simulink model "zrf_volt_1ant_8bit"  (R2019a)
settings: Solver=VariableStepAuto  StartTime=0.0  StopTime=10.0  RelTol=1e-3
undefined symbols (not defined in the file or in its folder): fft_stages
libraries: xbsIndex_r4 x8883, casper_library_misc x68, xps_library x15, casper_library_sources x8, casper_library_delays x2, casper_library_scopes x2
(part 2 of 97)

== system zrf_volt_1ant_8bit/HTG_ZRF16 ==

== system zrf_volt_1ant_8bit/adc_rstn ==
  convert1_1 : DataTypeConversion  OutDataTypeStr=fixdt('ufix1_En0')  LockScale=on
  convert2_1 : DataTypeConversion  OutDataTypeStr=fixdt('ufix1_En0')  ConvertRealWorld=Stored Integer (SI)  LockScale=on
  gain_1 : Gain
  io_delay : xbsIndex_r4/Delay  rst=off  infoeditControl=Selection of Reset will increase slice count due to use of real FFs and instead of SRLs  en=off  latency=0  reg_retiming=on  dbl_ovrd=off  block_type=delay
  sim_1 : Constant  Value=0
  slice_reg : xbsIndex_r4/Slice  nbits=1  boolean_output=on  mode=Lower Bit Location + Width  bit1=0  base1=MSB of Input  bit0=0  base0=LSB of Input  dbl_ovrd=off  block_type=slice
  zrf_volt_1ant_8bit_adc_rstn_user_data_out : xbsIndex_r4/Gateway In  gui_display_data_type=Fixed-point  arith_type=Unsigned  n_bits=32  bin_pt=0  preci_type=Single  exp_width=8  frac_width=24  rows=1  columns=1  quantization="Round  (unbiased: +/- Inf)"  overflow=Saturate  period=1  UseAsADC=off  ADCChannel='1'  interface=None  automatic_assignment=on  address_offset=hex2dec('00')  intf_name=''  intf_description=''  default_value=0  timing_constraint=None  locs_specified=off  LOCs={}  io_standard={}  inherit_from_input=off  hdl_port=on  dbl_ovrd=off  block_type=gatewayin
  in_reg : Outport
  wires:
  zrf_volt_1ant_8bit_adc_rstn_user_data_out/1 -> io_delay/1
  sim_1/1 -> convert1_1/1
  convert1_1/1 -> convert2_1/1
  convert2_1/1 -> gain_1/1
  gain_1/1 -> zrf_volt_1ant_8bit_adc_rstn_user_data_out/1
  io_delay/1 -> slice_reg/1
  slice_reg/1 -> in_reg/1

== system zrf_volt_1ant_8bit/byte_flip ==
  din : Inport
  join : Subsystem  AncestorBlock=casper_library_flow_control/bus_create  mask(bus_create){inputNum=64}
      mask prompts: inputNum "Number of inputs:"
      mask init:
      | bus_create_init(gcb,...
      |     'inputNum', inputNum);
  reinterpret : xbsIndex_r4/Reinterpret  force_arith_type=on  arith_type=Unsigned  force_bin_pt=on  bin_pt=0  block_type=reinterpret
  reinterpret_out : xbsIndex_r4/Reinterpret  force_arith_type=on  arith_type=Unsigned  force_bin_pt=on  bin_pt=0  block_type=reinterpret
  split : Subsystem  AncestorBlock=casper_library_flow_control/bus_expand  mask(bus_expand){mode=divisions of arbitrary size, outputNum=1, outputWidth=[8 8 8 8 8 8 8 8 8 8 8 8 8 8 8 8 8 8 8 8 8 8 8 8 8 8 8 8 8 8 8 8 8 8 8 8 8 8 8 8 8 8 8 8 8 8 8 8 8 8 8 8 8 8 8 8 8 8 8 8 8 8 8 8], outputBinaryPt=[0 0 0 0 0 0 0 0 0 0 0 0 0 0 0 0 0 0 0 0 0 0 0 0 0 0 0 0 0 0 0 0 0 0 0 0 0 0 0 0 0 0 0 0 0 0 0 0 0 0 0 0 0 0 0 0 0 0 0 0 0 0 0 0], outputArithmeticType=[0 0 0 0 0 0 0 0 0 0 0 0 0 0 0 0 0 0 0 0 0 0 0 0 0 0 0 0 0 0 0 0 0 0 0 0 0 0 0 0 0 0 0 0 0 0 0 0 0 0 0 0 0 0 0 0 0 0 0 0 0 0 0 0], show_format=off, outputToWorkspace=off, variablePrefix=out, outputToModelAsWell=on}
      mask prompts: outputNum "Number of outputs:"; outputWidth "Output width [msb ... lsb]:"; outputBinaryPt "Output binary point position [msb ... lsb]:"; outputArithmeticType "Output arithmetic type (ufix=0, fix=1, bool=2) [msb ... lsb]:"; show_format "Print format string?"; outputToWorkspace "Output to workspace?"; variablePrefix "Variable name prefix:"; outputToModelAsWell "Output to model as well?"
      mask help:
      | Expands a 'bus' made using a bus_create or Xilinx
      | concat block.
      | The input will be divided into the specified number
      | of outputs with the specified arithmetic types.
      | Divisions are made from most significant bit.
      mask init:
      | bus_expand_init(gcb,...
      |     'mode', mode, ...
      |     'outputNum', outputNum, ...
      |     'outputWidth', outputWidth, ...
      |     'outputBinaryPt', outputBinaryPt, ...
      |     'outputArithmeticType', outputArithmeticType, ...
      |     'show_format', show_format, ...
      |     'outputToWorkspace', outputToWorkspace, ...
      |     'variablePrefix', variablePrefix, ...
      |     'outputToModelAsWell', outputToModelAsWell);
      settings: AttributesFormatString=64 outputs
      mask TypeOptions mode: divisions of equal size | divisions of arbitrary size
      mask Callback mode: bus_expand_callback();
      mask Callback outputWidth: bus_expand_callback();
      mask Callback outputToWorkspace: bus_expand_callback();
  dout : Outport
  wires:
  reinterpret_out/1 -> dout/1
  din/1 -> reinterpret/1
  reinterpret/1 -> split/1(bus_in)
  join/1(bus_out) -> reinterpret_out/1
  split/64(lsb_out1) -> join/1(in1)
  split/63(out2) -> join/2(in2)
  split/62(out3) -> join/3(in3)
  split/61(out4) -> join/4(in4)
  split/60(out5) -> join/5(in5)
  split/59(out6) -> join/6(in6)
  split/58(out7) -> join/7(in7)
  split/57(out8) -> join/8(in8)
  split/56(out9) -> join/9(in9)
  split/55(out10) -> join/10(in10)
  split/54(out11) -> join/11(in11)
  split/53(out12) -> join/12(in12)
  split/52(out13) -> join/13(in13)
  split/51(out14) -> join/14(in14)
  split/50(out15) -> join/15(in15)
  split/49(out16) -> join/16(in16)
  split/48(out17) -> join/17(in17)
  split/47(out18) -> join/18(in18)
  split/46(out19) -> join/19(in19)
  split/45(out20) -> join/20(in20)
  split/44(out21) -> join/21(in21)
  split/43(out22) -> join/22(in22)
  split/42(out23) -> join/23(in23)
  split/41(out24) -> join/24(in24)
  split/40(out25) -> join/25(in25)
  split/39(out26) -> join/26(in26)
  split/38(out27) -> join/27(in27)
  split/37(out28) -> join/28(in28)
  split/36(out29) -> join/29(in29)
  split/35(out30) -> join/30(in30)
  split/34(out31) -> join/31(in31)
  split/33(out32) -> join/32(in32)
  split/32(out33) -> join/33(in33)
  split/31(out34) -> join/34(in34)
  split/30(out35) -> join/35(in35)
  split/29(out36) -> join/36(in36)
  split/28(out37) -> join/37(in37)
  split/27(out38) -> join/38(in38)
  split/26(out39) -> join/39(in39)
  split/25(out40) -> join/40(in40)
  split/24(out41) -> join/41(in41)
  split/23(out42) -> join/42(in42)
  split/22(out43) -> join/43(in43)
  split/21(out44) -> join/44(in44)
  split/20(out45) -> join/45(in45)
  split/19(out46) -> join/46(in46)
  split/18(out47) -> join/47(in47)
  split/17(out48) -> join/48(in48)
  split/16(out49) -> join/49(in49)
  split/15(out50) -> join/50(in50)
  split/14(out51) -> join/51(in51)
  split/13(out52) -> join/52(in52)
  split/12(out53) -> join/53(in53)
  split/11(out54) -> join/54(in54)
  split/10(out55) -> join/55(in55)
  split/9(out56) -> join/56(in56)
  split/8(out57) -> join/57(in57)
  split/7(out58) -> join/58(in58)
  split/6(out59) -> join/59(in59)
  split/5(out60) -> join/60(in60)
  split/4(out61) -> join/61(in61)
  split/3(out62) -> join/62(in62)
  split/2(out63) -> join/63(in63)
  split/1(msb_out64) -> join/64(in64)

== system zrf_volt_1ant_8bit/byte_flip1 ==
  din : Inport
  join : Subsystem  AncestorBlock=casper_library_flow_control/bus_create  mask(bus_create){inputNum=64}
      mask prompts: inputNum "Number of inputs:"
      mask init:
      | bus_create_init(gcb,...
      |     'inputNum', inputNum);
  reinterpret : xbsIndex_r4/Reinterpret  force_arith_type=on  arith_type=Unsigned  force_bin_pt=on  bin_pt=0  block_type=reinterpret
  reinterpret_out : xbsIndex_r4/Reinterpret  force_arith_type=on  arith_type=Unsigned  force_bin_pt=on  bin_pt=0  block_type=reinterpret
  split : Subsystem  AncestorBlock=casper_library_flow_control/bus_expand  mask(bus_expand){mode=divisions of arbitrary size, outputNum=1, outputWidth=[8 8 8 8 8 8 8 8 8 8 8 8 8 8 8 8 8 8 8 8 8 8 8 8 8 8 8 8 8 8 8 8 8 8 8 8 8 8 8 8 8 8 8 8 8 8 8 8 8 8 8 8 8 8 8 8 8 8 8 8 8 8 8 8], outputBinaryPt=[0 0 0 0 0 0 0 0 0 0 0 0 0 0 0 0 0 0 0 0 0 0 0 0 0 0 0 0 0 0 0 0 0 0 0 0 0 0 0 0 0 0 0 0 0 0 0 0 0 0 0 0 0 0 0 0 0 0 0 0 0 0 0 0], outputArithmeticType=[0 0 0 0 0 0 0 0 0 0 0 0 0 0 0 0 0 0 0 0 0 0 0 0 0 0 0 0 0 0 0 0 0 0 0 0 0 0 0 0 0 0 0 0 0 0 0 0 0 0 0 0 0 0 0 0 0 0 0 0 0 0 0 0], show_format=off, outputToWorkspace=off, variablePrefix=out, outputToModelAsWell=on}
      mask prompts: outputNum "Number of outputs:"; outputWidth "Output width [msb ... lsb]:"; outputBinaryPt "Output binary point position [msb ... lsb]:"; outputArithmeticType "Output arithmetic type (ufix=0, fix=1, bool=2) [msb ... lsb]:"; show_format "Print format string?"; outputToWorkspace "Output to workspace?"; variablePrefix "Variable name prefix:"; outputToModelAsWell "Output to model as well?"
      mask help:
      | Expands a 'bus' made using a bus_create or Xilinx
      | concat block.
      | The input will be divided into the specified number
      | of outputs with the specified arithmetic types.
      | Divisions are made from most significant bit.
      mask init: same as zrf_volt_1ant_8bit/byte_flip/split
      settings: AttributesFormatString=64 outputs
      mask TypeOptions mode: divisions of equal size | divisions of arbitrary size
      mask Callback mode: bus_expand_callback();
      mask Callback outputWidth: bus_expand_callback();
      mask Callback outputToWorkspace: bus_expand_callback();
  dout : Outport
  wires:
  split/1(msb_out64) -> join/64(in64)
  split/2(out63) -> join/63(in63)
  split/3(out62) -> join/62(in62)
  split/4(out61) -> join/61(in61)
  split/5(out60) -> join/60(in60)
  split/6(out59) -> join/59(in59)
  split/7(out58) -> join/58(in58)
  split/8(out57) -> join/57(in57)
  split/9(out56) -> join/56(in56)
  split/10(out55) -> join/55(in55)
  split/11(out54) -> join/54(in54)
  split/12(out53) -> join/53(in53)
  split/13(out52) -> join/52(in52)
  split/14(out51) -> join/51(in51)
  split/15(out50) -> join/50(in50)
  split/16(out49) -> join/49(in49)
  split/17(out48) -> join/48(in48)
  split/18(out47) -> join/47(in47)
  split/19(out46) -> join/46(in46)
  split/20(out45) -> join/45(in45)
  split/21(out44) -> join/44(in44)
  split/22(out43) -> join/43(in43)
  split/23(out42) -> join/42(in42)
  split/24(out41) -> join/41(in41)
  split/25(out40) -> join/40(in40)
  split/26(out39) -> join/39(in39)
  split/27(out38) -> join/38(in38)
  split/28(out37) -> join/37(in37)
  split/29(out36) -> join/36(in36)
  split/30(out35) -> join/35(in35)
  split/31(out34) -> join/34(in34)
  split/32(out33) -> join/33(in33)
  split/33(out32) -> join/32(in32)
  split/34(out31) -> join/31(in31)
  split/35(out30) -> join/30(in30)
  split/36(out29) -> join/29(in29)
  split/37(out28) -> join/28(in28)
  split/38(out27) -> join/27(in27)
  split/39(out26) -> join/26(in26)
  split/40(out25) -> join/25(in25)
  split/41(out24) -> join/24(in24)
  split/42(out23) -> join/23(in23)
  split/43(out22) -> join/22(in22)
  split/44(out21) -> join/21(in21)
  split/45(out20) -> join/20(in20)
  split/46(out19) -> join/19(in19)
  split/47(out18) -> join/18(in18)
  split/48(out17) -> join/17(in17)
  split/49(out16) -> join/16(in16)
  split/50(out15) -> join/15(in15)
  split/51(out14) -> join/14(in14)
  split/52(out13) -> join/13(in13)
  split/53(out12) -> join/12(in12)
  split/54(out11) -> join/11(in11)
  split/55(out10) -> join/10(in10)
  split/56(out9) -> join/9(in9)
  split/57(out8) -> join/8(in8)
  split/58(out7) -> join/7(in7)
  split/59(out6) -> join/6(in6)
  split/60(out5) -> join/5(in5)
  split/61(out4) -> join/4(in4)
  split/62(out3) -> join/3(in3)
  split/63(out2) -> join/2(in2)
  split/64(lsb_out1) -> join/1(in1)
  join/1(bus_out) -> reinterpret_out/1
  reinterpret/1 -> split/1(bus_in)
  din/1 -> reinterpret/1
  reinterpret_out/1 -> dout/1

== system zrf_volt_1ant_8bit/chan_reorder0 ==
  note: MANUALLY CHANGE BUFFER TO ULTRARAM
  note: output:
      | 4 ants x 2048 chans x [16 time x 2 pols]
      |
      | 8k clocks for complete cycle
  note: Use this programmable
      | map to mess with the channel
      | ordering.
      |
      | This lets us interleave channels we want to send, with channels
      | we don't care about, allowing the data rate to be kept below 10Gb/s
      |
      | Input is 4 channels x 2 pols in parallel.
      | Over 1024 clocks we get a full spectrum for these inputs.
  note: Reorder each parallel 64 bits to combine polarizations:
      |
      | order is now (for each of 4 antenna streams):
      |
      | serial_chans (512) x parallel_chans (4) x pols (2)
  note: reorder serial channels
      | so channels which we don't care about
      | can be placed in convenient
      | place to facilitate inter-packet gaps
  note: input: 16 times x 128 chans x 4 ants x 16 chans(parallel) x 2 pols
      |
      | output:
      | 4 ants x 128 chans x 16 times x 16 chans (parallel) x 2 pols
  note: Only allow one sync after MRST.
      | This is because we don't know the appropriate
      | reorder orders for non-double-buffered runtime-configuratble
      | reorders
  note: Merge streams into 512 bit bus:
      |
      | order is now:
      |
      | serial_chans (128) x 4 ants x parallel_chans (16) x pols (2)
  sync : Inport
  mrst : Inport  Port=2
  din0 : Inport  Port=3
  din1 : Inport  Port=4
  din2 : Inport  Port=5
  din3 : Inport  Port=6
  Concat : xbsIndex_r4/Concat  num_inputs=4  dbl_ovrd=off  block_type=concat
  Constant4 : xbsIndex_r4/Constant  const=1.0  gui_display_data_type=Boolean  arith_type=Boolean  n_bits=16  bin_pt=14  preci_type=Single  exp_width=8  frac_width=24  explicit_period=on  period=1  equ=P=C  opselect=C  inp2=PCIN>>17  opr=+  inp1=P  carry=CIN  dbl_ovrd=off  block_type=constant
  Inverter : xbsIndex_r4/Inverter  en=off  latency=0  dbl_ovrd=off  block_type=inv
  Logical : xbsIndex_r4/Logical  logical_function=AND  inputs=2  en=off  latency=0  precision=Full  arith_type=Unsigned  n_bits=16  bin_pt=0  align_bp=on  dbl_ovrd=off  block_type=logical
  Register : xbsIndex_r4/Register  init=0  rst=on  en=on  dbl_ovrd=off  block_type=register
  parallel_reorder0 : Subsystem
  parallel_reorder1 : Subsystem
  parallel_reorder2 : Subsystem
  parallel_reorder3 : Subsystem
  reorder2 : Subsystem  AncestorBlock=casper_library_reorder/reorder  mask(reorder){map=reshape(permute(reshape([0:512*16 - 1], 512, 16), [2,1]), 512*16, 1), n_bits=512, n_inputs=1, bram_latency=3, map_latency=1, fanout_latency=0, double_buffer=0, bram_map=on, software_controlled=off}
      mask prompts: map "Output Order:"; n_bits "Data width in"; n_inputs "Number of inputs"; bram_latency "BRAM Latency"; map_latency "Map Latency"; fanout_latency "Fanout latency"; double_buffer "Double Buffer"; bram_map "Use BlockRAM for Map"; software_controlled "Use runtime software control"
      mask init:
      | reorder_init(gcb, ...
      |     'map', map, ...
      |     'n_bits', n_bits, ...
      |     'n_inputs', n_inputs, ...
      |     'bram_latency', bram_latency, ...
      |     'map_latency', map_latency, ...
      |     'fanout_latency', fanout_latency, ...
      |     'double_buffer', double_buffer, ...
      |     'bram_map', bram_map, ...
      |     'software_controlled', software_controlled);
      settings: AttributesFormatString=order=13
      mask Help: eval('xlWeb(''http://casper.berkeley.edu/wiki/Reorder'')')
  skip_c_t_transpose : Subsystem  Tag=xps:sw_reg  AncestorBlock=xps_library/Memory/software_register  mask(swreg){io_dir=From Processor, io_delay=0, init_val=0, sample_period=1, names=reg, bitwidths=1, bin_pts=0, arith_types=0, sim_port=on, show_format=on}
      mask prompts: io_dir "I/O direction"; io_delay "I/O delay"; init_val "Initial Value"; sample_period "Sample period"; names "Bitfield names [msb...lsb]"; bitwidths "Bitfield widths"; bin_pts "Bitfield binary pts"; arith_types "Bitfield types, ufix=0, fix=1, bool=2"; sim_port "Provide sim input/output?"; show_format "Print format string?"
      mask help: A 32-bit software-accessible register. Can be divided into bitfields of varying widths and types using the fields in the block mask.
      mask init:
      | swreg_init(gcb)
      settings: AttributesFormatString=1input:uf1.0 = 1 bits
      mask TypeOptions io_dir: To Processor | From Processor
      mask Callback io_dir:
      | mask_enables = get_param(gcb, 'MaskEnables');
      | mask_names = get_param(gcb, 'MaskNames');
      | if strcmp(get_param(gcb, 'io_dir'), 'To Processor'),
      |     mask_enables{ismember(mask_names, 'sample_period')} = 'off';
      | else
      |     mask_enables{ismember(mask_names, 'sample_period')} = 'on';
      | end
      | set_param(gcb, 'MaskEnables', mask_enables);
      mask DialogControl ParameterTabVar0 Prompt: Setup
  square_transposer : Subsystem  AncestorBlock=casper_library_reorder/square_transposer  mask(square_transposer){n_inputs=2, async=off}
      mask prompts: n_inputs "Number of inputs (2^?):"; async "Aynchronus operation"
      mask init:
      | square_transposer_init(gcb,...
      |     'n_inputs', n_inputs, ...
      |     'async', async);
      settings: AttributesFormatString=n_inputs=2
      mask Help: eval('xlWeb(''http://casper.berkeley.edu/wiki/Square_transposer'')')
  transpose_t_c : Subsystem
  sync_out : Outport
  dout0 : Outport  Port=2
  wires:
  skip_c_t_transpose/1(in_reg) -> transpose_t_c/3(bypass)
  transpose_t_c/2(dout) -> dout0/1
  transpose_t_c/1(sync_out) -> sync_out/1
  reorder2/3(dout0) -> transpose_t_c/2(din)
  reorder2/1(sync_out) -> transpose_t_c/1(sync)
  Inverter/1 -> Logical/1
  Register/1 -> Inverter/1
  mrst/1 -> Register/2
  Constant4/1 -> reorder2/2(en)
  Logical/1 -> square_transposer/1(sync)
  sync/1 -> Register/3, Register/1, Logical/2
  din0/1 -> parallel_reorder0/1(din)
  parallel_reorder3/1(dout) -> square_transposer/5(in3)
  parallel_reorder2/1(dout) -> square_transposer/4(in2)
  parallel_reorder1/1(dout) -> square_transposer/3(in1)
  parallel_reorder0/1(dout) -> square_transposer/2(in0)
  square_transposer/1(sync_out) -> reorder2/1(sync)
  Concat/1 -> reorder2/3(din0)
  din1/1 -> parallel_reorder1/1(din)
  din2/1 -> parallel_reorder2/1(din)
  din3/1 -> parallel_reorder3/1(din)
  square_transposer/5(out3) -> Concat/4
  square_transposer/4(out2) -> Concat/3
  square_transposer/3(out1) -> Concat/2
  square_transposer/2(out0) -> Concat/1

== system zrf_volt_1ant_8bit/chan_reorder1 ==
  note: Merge streams into 512 bit bus:
      |
      | order is now:
      |
      | serial_chans (128) x 4 ants x parallel_chans (16) x pols (2)
  note: Only allow one sync after MRST.
      | This is because we don't know the appropriate
      | reorder orders for non-double-buffered runtime-configuratble
      | reorders
  note: input: 16 times x 128 chans x 4 ants x 16 chans(parallel) x 2 pols
      |
      | output:
      | 4 ants x 128 chans x 16 times x 16 chans (parallel) x 2 pols
  note: reorder serial channels
      | so channels which we don't care about
      | can be placed in convenient
      | place to facilitate inter-packet gaps
  note: Reorder each parallel 64 bits to combine polarizations:
      |
      | order is now (for each of 4 antenna streams):
      |
      | serial_chans (512) x parallel_chans (4) x pols (2)
  note: Use this programmable
      | map to mess with the channel
      | ordering.
      |
      | This lets us interleave channels we want to send, with channels
      | we don't care about, allowing the data rate to be kept below 10Gb/s
      |
      | Input is 4 channels x 2 pols in parallel.
      | Over 1024 clocks we get a full spectrum for these inputs.
  note: output:
      | 4 ants x 2048 chans x [16 time x 2 pols]
      |
      | 8k clocks for complete cycle
  note: MANUALLY CHANGE BUFFER TO ULTRARAM
  sync : Inport
  mrst : Inport  Port=2
  din0 : Inport  Port=3
  din1 : Inport  Port=4
  din2 : Inport  Port=5
  din3 : Inport  Port=6
  Concat : xbsIndex_r4/Concat  num_inputs=4  dbl_ovrd=off  block_type=concat
  Constant4 : xbsIndex_r4/Constant  const=1.0  gui_display_data_type=Boolean  arith_type=Boolean  n_bits=16  bin_pt=14  preci_type=Single  exp_width=8  frac_width=24  explicit_period=on  period=1  equ=P=C  opselect=C  inp2=PCIN>>17  opr=+  inp1=P  carry=CIN  dbl_ovrd=off  block_type=constant
  Inverter : xbsIndex_r4/Inverter  en=off  latency=0  dbl_ovrd=off  block_type=inv
  Logical : xbsIndex_r4/Logical  logical_function=AND  inputs=2  en=off  latency=0  precision=Full  arith_type=Unsigned  n_bits=16  bin_pt=0  align_bp=on  dbl_ovrd=off  block_type=logical
  Register : xbsIndex_r4/Register  init=0  rst=on  en=on  dbl_ovrd=off  block_type=register
  parallel_reorder0 : Subsystem
  parallel_reorder1 : Subsystem
  parallel_reorder2 : Subsystem
  parallel_reorder3 : Subsystem
  reorder2 : Subsystem  AncestorBlock=casper_library_reorder/reorder  mask(reorder){map=reshape(permute(reshape([0:512*16 - 1], 512, 16), [2,1]), 512*16, 1), n_bits=512, n_inputs=1, bram_latency=3, map_latency=1, fanout_latency=0, double_buffer=0, bram_map=on, software_controlled=off}
      mask prompts: map "Output Order:"; n_bits "Data width in"; n_inputs "Number of inputs"; bram_latency "BRAM Latency"; map_latency "Map Latency"; fanout_latency "Fanout latency"; double_buffer "Double Buffer"; bram_map "Use BlockRAM for Map"; software_controlled "Use runtime software control"
      mask init: same as zrf_volt_1ant_8bit/chan_reorder0/reorder2
      settings: AttributesFormatString=order=13
      mask Help: eval('xlWeb(''http://casper.berkeley.edu/wiki/Reorder'')')
  skip_c_t_transpose : Subsystem  Tag=xps:sw_reg  AncestorBlock=xps_library/Memory/software_register  mask(swreg){io_dir=From Processor, io_delay=0, init_val=0, sample_period=1, names=reg, bitwidths=1, bin_pts=0, arith_types=0, sim_port=on, show_format=on}
      mask prompts: io_dir "I/O direction"; io_delay "I/O delay"; init_val "Initial Value"; sample_period "Sample period"; names "Bitfield names [msb...lsb]"; bitwidths "Bitfield widths"; bin_pts "Bitfield binary pts"; arith_types "Bitfield types, ufix=0, fix=1, bool=2"; sim_port "Provide sim input/output?"; show_format "Print format string?"
      mask help: A 32-bit software-accessible register. Can be divided into bitfields of varying widths and types using the fields in the block mask.
      mask init:
      | swreg_init(gcb)
      settings: AttributesFormatString=1input:uf1.0 = 1 bits
      mask TypeOptions io_dir: To Processor | From Processor
      mask Callback io_dir:
      | mask_enables = get_param(gcb, 'MaskEnables');
      | mask_names = get_param(gcb, 'MaskNames');
      | if strcmp(get_param(gcb, 'io_dir'), 'To Processor'),
      |     mask_enables{ismember(mask_names, 'sample_period')} = 'off';
      | else
      |     mask_enables{ismember(mask_names, 'sample_period')} = 'on';
      | end
      | set_param(gcb, 'MaskEnables', mask_enables);
      mask DialogControl ParameterTabVar0 Prompt: Setup
  square_transposer : Subsystem  AncestorBlock=casper_library_reorder/square_transposer  mask(square_transposer){n_inputs=2, async=off}
      mask prompts: n_inputs "Number of inputs (2^?):"; async "Aynchronus operation"
      mask init:
      | square_transposer_init(gcb,...
      |     'n_inputs', n_inputs, ...
      |     'async', async);
      settings: AttributesFormatString=n_inputs=2
      mask Help: eval('xlWeb(''http://casper.berkeley.edu/wiki/Square_transposer'')')
  transpose_t_c : Subsystem
  sync_out : Outport
  dout0 : Outport  Port=2
  wires:
  square_transposer/2(out0) -> Concat/1
  square_transposer/3(out1) -> Concat/2
  square_transposer/4(out2) -> Concat/3
  square_transposer/5(out3) -> Concat/4
  din3/1 -> parallel_reorder3/1(din)
  din2/1 -> parallel_reorder2/1(din)
  din1/1 -> parallel_reorder1/1(din)
  Concat/1 -> reorder2/3(din0)
  square_transposer/1(sync_out) -> reorder2/1(sync)
  parallel_reorder0/1(dout) -> square_transposer/2(in0)
  parallel_reorder1/1(dout) -> square_transposer/3(in1)
  parallel_reorder2/1(dout) -> square_transposer/4(in2)
  parallel_reorder3/1(dout) -> square_transposer/5(in3)
  din0/1 -> parallel_reorder0/1(din)
  sync/1 -> Logical/2, Register/1, Register/3
  Logical/1 -> square_transposer/1(sync)
  Constant4/1 -> reorder2/2(en)
  mrst/1 -> Register/2
  Register/1 -> Inverter/1
  Inverter/1 -> Logical/1
  reorder2/1(sync_out) -> transpose_t_c/1(sync)
  reorder2/3(dout0) -> transpose_t_c/2(din)
  transpose_t_c/1(sync_out) -> sync_out/1
  transpose_t_c/2(dout) -> dout0/1
  skip_c_t_transpose/1(in_reg) -> transpose_t_c/3(bypass)

== system zrf_volt_1ant_8bit/corr ==
  sync : Inport
  din : Inport  Port=2
  mrst : Inport  Port=3
  bus_create1 : Subsystem  AncestorBlock=casper_library_flow_control/bus_create  mask(bus_create){inputNum=4}
      mask prompts: inputNum "Number of inputs:"
      mask init:
      | bus_create_init(gcb,...
      |     'inputNum', inputNum);
  bus_expand : Subsystem  AncestorBlock=casper_library_flow_control/bus_expand  mask(bus_expand){mode=divisions of equal size, outputNum=2, outputWidth=25*2*4, outputBinaryPt=0, outputArithmeticType=0, show_format=off, outputToWorkspace=off, variablePrefix=out, outputToModelAsWell=on}
      mask prompts: outputNum "Number of outputs:"; outputWidth "Output width:"; outputBinaryPt "Output binary point position:"; outputArithmeticType "Output arithmetic type (ufix=0, fix=1, bool=2):"; show_format "Print format string?"; outputToWorkspace "Output to workspace?"; variablePrefix "Variable name prefix:"; outputToModelAsWell "Output to model as well?"
      mask help:
      | Expands a 'bus' made using a bus_create or Xilinx
      | concat block.
      | The input will be divided into the specified number
      | of outputs with the specified arithmetic types.
      | Divisions are made from most significant bit.
      mask init: same as zrf_volt_1ant_8bit/byte_flip/split
      settings: AttributesFormatString=2 outputs
      mask TypeOptions mode: divisions of equal size | divisions of arbitrary size
      mask Callback mode: bus_expand_callback();
      mask Callback outputWidth: bus_expand_callback();
      mask Callback outputToWorkspace: bus_expand_callback();
  bus_expand3 : Subsystem  AncestorBlock=casper_library_flow_control/bus_expand  mask(bus_expand){mode=divisions of equal size, outputNum=4, outputWidth=25*2, outputBinaryPt=0, outputArithmeticType=0, show_format=off, outputToWorkspace=off, variablePrefix=out, outputToModelAsWell=on}
      mask prompts: outputNum "Number of outputs:"; outputWidth "Output width:"; outputBinaryPt "Output binary point position:"; outputArithmeticType "Output arithmetic type (ufix=0, fix=1, bool=2):"; show_format "Print format string?"; outputToWorkspace "Output to workspace?"; variablePrefix "Variable name prefix:"; outputToModelAsWell "Output to model as well?"
      mask help:
      | Expands a 'bus' made using a bus_create or Xilinx
      | concat block.
      | The input will be divided into the specified number
      | of outputs with the specified arithmetic types.
      | Divisions are made from most significant bit.
      mask init: same as zrf_volt_1ant_8bit/byte_flip/split
      settings: AttributesFormatString=4 outputs
      mask TypeOptions mode: divisions of equal size | divisions of arbitrary size
      mask Callback mode: bus_expand_callback();
      mask Callback outputWidth: bus_expand_callback();
      mask Callback outputToWorkspace: bus_expand_callback();
  bus_expand4 : Subsystem  AncestorBlock=casper_library_flow_control/bus_expand  mask(bus_expand){mode=divisions of equal size, outputNum=4, outputWidth=25*2, outputBinaryPt=0, outputArithmeticType=0, show_format=off, outputToWorkspace=off, variablePrefix=out, outputToModelAsWell=on}
      mask prompts: outputNum "Number of outputs:"; outputWidth "Output width:"; outputBinaryPt "Output binary point position:"; outputArithmeticType "Output arithmetic type (ufix=0, fix=1, bool=2):"; show_format "Print format string?"; outputToWorkspace "Output to workspace?"; variablePrefix "Variable name prefix:"; outputToModelAsWell "Output to model as well?"
      mask help:
      | Expands a 'bus' made using a bus_create or Xilinx
      | concat block.
      | The input will be divided into the specified number
      | of outputs with the specified arithmetic types.
      | Divisions are made from most significant bit.
      mask init: same as zrf_volt_1ant_8bit/byte_flip/split
      settings: AttributesFormatString=4 outputs
      mask TypeOptions mode: divisions of equal size | divisions of arbitrary size
      mask Callback mode: bus_expand_callback();
      mask Callback outputWidth: bus_expand_callback();
      mask Callback outputToWorkspace: bus_expand_callback();
  crosspower_vacc : Subsystem  mask{bw=25, nchan=2^n_chan_bits, vacc_bw=64, vacc_bp=48}
      mask prompts: bw "Bitwidth in"; nchan "Number of channels"; vacc_bw "Vector accumulator output bitwidth"; vacc_bp "Vector accumulator output binary point"
  ss_vld_out : Outport
  ss_dout : Outport  Port=2
  wires:
  din/1 -> bus_expand/1(bus_in)
  bus_expand/1(msb_out2) -> [x]
  bus_expand/2(lsb_out1) -> [y]
  sync/1 -> [sync_in]
  mrst/1 -> [mrst_in]
  crosspower_vacc/2(xy0) -> [xy_0]
  crosspower_vacc/5(xy3) -> [xy_3]
  crosspower_vacc/4(xy2) -> [xy_2]
  crosspower_vacc/3(xy1) -> [xy_1]
  bus_expand3/1(msb_out4) -> crosspower_vacc/2(x0)
  bus_expand3/2(out3) -> crosspower_vacc/3(x1)
  bus_expand3/3(out2) -> crosspower_vacc/4(x2)
  bus_expand3/4(lsb_out1) -> crosspower_vacc/5(x3)
  bus_expand4/1(msb_out4) -> crosspower_vacc/6(y0)
  bus_expand4/2(out3) -> crosspower_vacc/7(y1)
  bus_expand4/3(out2) -> crosspower_vacc/8(y2)
  bus_expand4/4(lsb_out1) -> crosspower_vacc/9(y3)
  [vacc_vld] -> ss_vld_out/1
  bus_create1/1(bus_out) -> ss_dout/1
  [sync_in] -> crosspower_vacc/1(new_acc)
  [x] -> bus_expand3/1(bus_in)
  [y] -> bus_expand4/1(bus_in)
  [xy_0] -> bus_create1/1(in1)
  [xy_1] -> bus_create1/2(in2)
  [xy_2] -> bus_create1/3(in3)
  [xy_3] -> bus_create1/4(in4)
  crosspower_vacc/1(vld) -> [vacc_vld]

== system zrf_volt_1ant_8bit/corr_quant ==
  sync : Inport
  din : Inport  Port=2
  bus_expand : Subsystem  AncestorBlock=casper_library_flow_control/bus_expand  mask(bus_expand){mode=divisions of equal size, outputNum=2, outputWidth=4*2*4, outputBinaryPt=0, outputArithmeticType=0, show_format=off, outputToWorkspace=off, variablePrefix=out, outputToModelAsWell=on}
      mask prompts: outputNum "Number of outputs:"; outputWidth "Output width:"; outputBinaryPt "Output binary point position:"; outputArithmeticType "Output arithmetic type (ufix=0, fix=1, bool=2):"; show_format "Print format string?"; outputToWorkspace "Output to workspace?"; variablePrefix "Variable name prefix:"; outputToModelAsWell "Output to model as well?"
      mask help:
      | Expands a 'bus' made using a bus_create or Xilinx
      | concat block.
      | The input will be divided into the specified number
      | of outputs with the specified arithmetic types.
      | Divisions are made from most significant bit.
      mask init: same as zrf_volt_1ant_8bit/byte_flip/split
      settings: AttributesFormatString=2 outputs
      mask TypeOptions mode: divisions of equal size | divisions of arbitrary size
      mask Callback mode: bus_expand_callback();
      mask Callback outputWidth: bus_expand_callback();
      mask Callback outputToWorkspace: bus_expand_callback();
  bus_expand1 : Subsystem  AncestorBlock=casper_library_flow_control/bus_expand  mask(bus_expand){mode=divisions of equal size, outputNum=4, outputWidth=4*2, outputBinaryPt=0, outputArithmeticType=1, show_format=off, outputToWorkspace=off, variablePrefix=out, outputToModelAsWell=on}
      mask prompts: outputNum "Number of outputs:"; outputWidth "Output width:"; outputBinaryPt "Output binary point position:"; outputArithmeticType "Output arithmetic type (ufix=0, fix=1, bool=2):"; show_format "Print format string?"; outputToWorkspace "Output to workspace?"; variablePrefix "Variable name prefix:"; outputToModelAsWell "Output to model as well?"
      mask help:
      | Expands a 'bus' made using a bus_create or Xilinx
      | concat block.
      | The input will be divided into the specified number
      | of outputs with the specified arithmetic types.
      | Divisions are made from most significant bit.
      mask init: same as zrf_volt_1ant_8bit/byte_flip/split
      settings: AttributesFormatString=4 outputs
      mask TypeOptions mode: divisions of equal size | divisions of arbitrary size
      mask Callback mode: bus_expand_callback();
      mask Callback outputWidth: bus_expand_callback();
      mask Callback outputToWorkspace: bus_expand_callback();
  bus_expand2 : Subsystem  AncestorBlock=casper_library_flow_control/bus_expand  mask(bus_expand){mode=divisions of equal size, outputNum=4, outputWidth=4*2, outputBinaryPt=0, outputArithmeticType=1, show_format=off, outputToWorkspace=off, variablePrefix=out, outputToModelAsWell=on}
      mask prompts: outputNum "Number of outputs:"; outputWidth "Output width:"; outputBinaryPt "Output binary point position:"; outputArithmeticType "Output arithmetic type (ufix=0, fix=1, bool=2):"; show_format "Print format string?"; outputToWorkspace "Output to workspace?"; variablePrefix "Variable name prefix:"; outputToModelAsWell "Output to model as well?"
      mask help:
      | Expands a 'bus' made using a bus_create or Xilinx
      | concat block.
      | The input will be divided into the specified number
      | of outputs with the specified arithmetic types.
      | Divisions are made from most significant bit.
      mask init: same as zrf_volt_1ant_8bit/byte_flip/split
      settings: AttributesFormatString=4 outputs
      mask TypeOptions mode: divisions of equal size | divisions of arbitrary size
      mask Callback mode: bus_expand_callback();
      mask Callback outputWidth: bus_expand_callback();
      mask Callback outputToWorkspace: bus_expand_callback();
  power_vacc0 : Subsystem  mask{bw=8, nchan=2^n_chan_bits, vacc_bw=32, vacc_bp=14}
      mask prompts: bw "Bitwidth in"; nchan "Number of channels"; vacc_bw "Vector accumulator output bitwidth"; vacc_bp "Vector accumulator output binary point"
  power_vacc1 : Subsystem  mask{bw=8, nchan=2^n_chan_bits, vacc_bw=32, vacc_bp=14}
      mask prompts: bw "Bitwidth in"; nchan "Number of channels"; vacc_bw "Vector accumulator output bitwidth"; vacc_bp "Vector accumulator output binary point"
  vacc_ss : Subsystem  mask{n_chan_bits=n_chan_bits}
      mask prompts: n_chan_bits "Number of channels (2^?)"
      mask init:
      | ss0 = [gcb '/ss0']
      | %ss1 = [gcb '/ss1']
      | 
      | nsamples = num2str(n_chan_bits - 2);
      | 
      | set_param(ss0, 'nsamples', nsamples);
      | %set_param(ss1, 'nsamples', nsamples);
  wires:
  bus_expand2/4(lsb_out1) -> power_vacc1/5(in3)
  bus_expand2/3(out2) -> power_vacc1/4(in2)
  bus_expand2/2(out3) -> power_vacc1/3(in1)
  bus_expand2/1(msb_out4) -> power_vacc1/2(in0)
  bus_expand1/4(lsb_out1) -> power_vacc0/5(in3)
  bus_expand1/3(out2) -> power_vacc0/4(in2)
  bus_expand1/2(out3) -> power_vacc0/3(in1)
  bus_expand1/1(msb_out4) -> power_vacc0/2(in0)
  [yy_3] -> vacc_ss/9(yy3)
  [yy_2] -> vacc_ss/8(yy2)
  [yy_1] -> vacc_ss/7(yy1)
  [yy_0] -> vacc_ss/6(yy0)
  [xx_3] -> vacc_ss/5(xx3)
  [xx_2] -> vacc_ss/4(xx2)
  power_vacc1/5(out3) -> [yy_3]
  power_vacc1/4(out2) -> [yy_2]
  power_vacc1/3(out1) -> [yy_1]
  power_vacc1/2(out0) -> [yy_0]
  power_vacc0/5(out3) -> [xx_3]
  power_vacc0/4(out2) -> [xx_2]
  power_vacc0/3(out1) -> [xx_1]
  power_vacc0/2(out0) -> [xx_0]
  [xx_1] -> vacc_ss/3(xx1)
  [vacc_vld] -> vacc_ss/1(vld)
  [xx_0] -> vacc_ss/2(xx0)
  [y] -> bus_expand2/1(bus_in)
  sync/1 -> [sync_in]
  [sync_in] -> power_vacc1/1(new_acc)
  [x] -> bus_expand1/1(bus_in)
  bus_expand/2(lsb_out1) -> [y]
  bus_expand/1(msb_out2) -> [x]
  din/1 -> bus_expand/1(bus_in)
  power_vacc0/1(vld) -> [vacc_vld]
  [sync_in] -> power_vacc0/1(new_acc)

== system zrf_volt_1ant_8bit/edge_detect ==
  in : Inport
  Delay : xbsIndex_r4/Delay  rst=off  infoeditControl=Selection of Reset will increase slice count due to use of real FFs and instead of SRLs  en=off  latency=1  reg_retiming=off  dbl_ovrd=off  block_type=delay
      settings: xl_area=[0, 0, 0, 0, 0, 0, 0]
  Inverter : xbsIndex_r4/Inverter  en=off  latency=0  dbl_ovrd=off  block_type=inv
      settings: xl_area=[0, 0, 0, 0, 0, 0, 0]
  edge_op : xbsIndex_r4/Logical  logical_function=NOR  inputs=2  en=off  latency=0  precision=Full  arith_type=Unsigned  n_bits=8  bin_pt=2  align_bp=on  dbl_ovrd=off  block_type=logical
      settings: xl_area=[0, 0, 0, 0, 0, 0, 0]
  out : Outport
  wires:
  Inverter/1 -> edge_op/1
  edge_op/1 -> out/1
  in/1 -> Inverter/1, Delay/1
  Delay/1 -> edge_op/2

== system zrf_volt_1ant_8bit/eth0 ==
  data : Inport
  vld : Inport  Port=2
  eof : Inport  Port=3
  dest_ip : Inport  Port=4
  dest_port : Inport  Port=5
  byte_enable : Inport  Port=6
  Constant : xbsIndex_r4/Constant  const=0  gui_display_data_type=Boolean  arith_type=Boolean  n_bits=1  bin_pt=0  preci_type=Single  exp_width=8  frac_width=24  explicit_period=on  period=1  equ=P=C  opselect=C  inp2=PCIN>>17  opr=+  inp1=P  carry=CIN  dbl_ovrd=off  block_type=constant
  Constant1 : xbsIndex_r4/Constant  const=0  gui_display_data_type=Boolean  arith_type=Boolean  n_bits=1  bin_pt=0  preci_type=Single  exp_width=8  frac_width=24  explicit_period=on  period=1  equ=P=C  opselect=C  inp2=PCIN>>17  opr=+  inp1=P  carry=CIN  dbl_ovrd=off  block_type=constant
  Constant2 : xbsIndex_r4/Constant  const=1  gui_display_data_type=Fixed-point  arith_type=Unsigned  n_bits=1  bin_pt=0  preci_type=Single  exp_width=8  frac_width=24  explicit_period=on  period=1  equ=P=C  opselect=C  inp2=PCIN>>17  opr=+  inp1=P  carry=CIN  dbl_ovrd=off  block_type=constant
  Constant3 : xbsIndex_r4/Constant  const=0  gui_display_data_type=Fixed-point  arith_type=Unsigned  n_bits=1  bin_pt=0  preci_type=Single  exp_width=8  frac_width=24  explicit_period=on  period=1  equ=P=C  opselect=C  inp2=PCIN>>17  opr=+  inp1=P  carry=CIN  dbl_ovrd=off  block_type=constant
  Delay : xbsIndex_r4/Delay  rst=off  infoeditControl=Selection of Reset will increase slice count due to use of real FFs and instead of SRLs  en=off  latency=1  reg_retiming=off  dbl_ovrd=off  block_type=delay
  Logical : xbsIndex_r4/Logical  logical_function=AND  inputs=2  en=off  latency=0  precision=Full  arith_type=Unsigned  n_bits=16  bin_pt=0  align_bp=on  dbl_ovrd=off  block_type=logical
  Register : xbsIndex_r4/Register  init=0  rst=off  en=on  dbl_ovrd=off  block_type=register
  Slice : xbsIndex_r4/Slice  nbits=1  boolean_output=on  mode=Lower Bit Location + Width  bit1=0  base1=MSB of Input  bit0=0  base0=LSB of Input  dbl_ovrd=off  block_type=slice
  Slice1 : xbsIndex_r4/Slice  nbits=1  boolean_output=on  mode=Lower Bit Location + Width  bit1=0  base1=MSB of Input  bit0=1  base0=LSB of Input  dbl_ovrd=off  block_type=slice
  Slice2 : xbsIndex_r4/Slice  nbits=16  boolean_output=off  mode=Lower Bit Location + Width  bit1=0  base1=MSB of Input  bit0=2  base0=LSB of Input  dbl_ovrd=off  block_type=slice
  Slice3 : xbsIndex_r4/Slice  nbits=1  boolean_output=on  mode=Lower Bit Location + Width  bit1=0  base1=MSB of Input  bit0=2+16  base0=LSB of Input  dbl_ovrd=off  block_type=slice
  ctrl : Subsystem  Tag=xps:sw_reg  AncestorBlock=xps_library/Memory/software_register  mask(swreg){io_dir=From Processor, io_delay=0, init_val=0, sample_period=1, names=reg, bitwidths=32, bin_pts=0, arith_types=0, sim_port=on, show_format=off}
      mask prompts: io_dir "I/O direction"; io_delay "I/O delay"; init_val "Initial Value"; sample_period "Sample period"; names "Bitfield names [msb...lsb]"; bitwidths "Bitfield widths"; bin_pts "Bitfield binary pts"; arith_types "Bitfield types, ufix=0, fix=1, bool=2"; sim_port "Provide sim input/output?"; show_format "Print format string?"
      mask help: A 32-bit software-accessible register. Can be divided into bitfields of varying widths and types using the fields in the block mask.
      mask init:
      | swreg_init(gcb)
      settings: AttributesFormatString=1input
      mask TypeOptions io_dir: To Processor | From Processor
      mask Callback io_dir:
      | mask_enables = get_param(gcb, 'MaskEnables');
      | mask_names = get_param(gcb, 'MaskNames');
      | if strcmp(get_param(gcb, 'io_dir'), 'To Processor'),
      |     mask_enables{ismember(mask_names, 'sample_period')} = 'off';
      | else
      |     mask_enables{ismember(mask_names, 'sample_period')} = 'on';
      | end
      | set_param(gcb, 'MaskEnables', mask_enables);
      mask DialogControl ParameterTabVar0 Prompt: Setup
  lpmode_gpio : xps_library/IO/gpio  Tag=xps:gpio  io_group_params_forwarded=off  io_group=ROACH:led  io_group_real=custom  io_group_custom=qsfp_lpmode  io_dir=out  arith_type=Unsigned  bitwidth=1  bin_pt=0  bit_index=[0]  sample_period=1  use_single_ended=off  use_ddr=off  reg_iob=on  reg_clk_phase=0  termination=None
      settings: SourceProductName=CASPER XPS Blockset
  onehundred_gbe : Subsystem  Tag=xps:onehundred_gbe  AncestorBlock=xps_library/IO/onehundred_gbe  mask(forty_gbe){flavour=cx4, slot=1, port_r1=0, port_r2_cx4=0, port_r2_sfpp=0, port=0, rx_dist_ram=on, large_frames=on, input_pipeline_delay=0, show_param=on, pre_emph_r2=0.74, pre_emph=3, post_emph_r2=0.18, rxeqmix_r2=7, swing_r2=940, swing=800, fab_en=on, fab_mac=hex2dec('123456780000'), fab_ip=192*(2^24) + 168*(2^16) + 5*(2^8) + 20*(2^0), fab_udp=10000, fab_gate=1, cpu_rx_en=on, cpu_tx_en=on, ttl=hex2dec('FF'), promisc_mode=off, debug_ctr_width=16, debug_en_all=off, debug_dis_all=off, txctr=off, txerrctr=off, txerrctr_len=100, txofctr=off, txfullctr=off, txvldctr=off, txsnaplen=0 - no snap, rxctr=off, rxerrctr=off, rxerrctr_len=100, rxofctr=off, rxbadctr=off, rxvldctr=off, rxeofctr=off, rxsnaplen=0 - no snap, rxsrcip=off, rxdstip=off}
      mask prompts: flavour "Mezzanine card flavour"; slot "Card slot"; port_r1 "Port"; port_r2_cx4 "Port"; port_r2_sfpp "Port"; rx_dist_ram "Shallow RX Fifo (Beware overruns!)"; large_frames "Enable Large TX Frames (8k+512)"; input_pipeline_delay "Incoming pipeline delay"; show_param "---------------------- Show Implementation Parameters -----------------------------------------------------------------------------------"; pre_emph_r2 "Pre-emphasis (dB)"; pre_emph "Pre-emphasis"; post_emph_r2 "Post-emphasis (dB)"; rxeqmix_r2 "Receive equalisation"; swing_r2 "Driver Swing Control (mVppd)"; swing "Differential swing"; fab_en "Enable fabric on startup"; fab_mac "Fabric MAC Address"; fab_ip "Fabric IP Address"; fab_udp "Fabric UDP Port"; fab_gate "Fabric Gateway"; cpu_rx_en "Enable CPU RX"; cpu_tx_en "Enable CPU TX"; promisc_mode "Promiscuous mode"; debug_ctr_width "Debug counter width"; debug_en_all "Enable all counters (overrides individual settings)"; debug_dis_all "Disable all counters (overrides individual settings)"; txctr "TX - core_txctr"; txerrctr "TX packet length error - core_txerrctr"; txerrctr_len "-- expected TX packet length"; txofctr "TX overflow - core_txofctr"; txfullctr "TX full - core_txfullctr"; txvldctr "TX valid cycle - core_txvldctr"; txsnaplen "TX snapshot length"; rxctr "RX - core_rxctr"; rxerrctr "RX packet length error - core_rxerrctr"; rxerrctr_len "-- expected RX packet length"; rxofctr "RX overflow - core_rxofctr"; rxbadctr "RX bad - core_rxbadctr"; rxvldctr "RX valid cycle - core_rxvldctr"; rxeofctr "RX eof - core_rxeofctr"; rxsnaplen "RX snapshot length"; rxsrcip "RX snapshot - include source IPs"; rxdstip "RX snapshot - include destination IPs"
      mask help: This block sends and receives UDP frames (packets). It accepts a 64 bit wide data stream with user-determined frame breaks. The data stream is wrapped in a UDP frame for transmission. Incoming UDP packets are unwrapped and the data presented as a 64 bit wide stream.
      mask init:
      | temp = eval(get_param(gcb, 'debug_ctr_width'));
      | if temp <= 0,
      |     error('Debug counters cannot be <= zero.');
      | end
      | onehundred_gbe_mask(gcb)
      settings: AttributesFormatString=incoming_latency=0
      mask TypeOptions flavour: sfp+ | cx4
      mask Callback flavour: forty_gbe_callback
      mask TypeOptions slot: 0 | 1
      mask TypeOptions port_r1: 0 | 1 | 2 | 3
      mask TypeOptions port_r2_cx4: 0 | 1 | 2
      mask TypeOptions port_r2_sfpp: 0 | 1 | 2 | 3
      mask TypeOptions port: 0 | 1 | 2 | 3
      mask Callback show_param: forty_gbe_callback
      mask TypeOptions pre_emph_r2: 0.15 | 0.3 | 0.45 | 0.61 | 0.74 | 0.91 | 1.07 | 1.25 | 1.36 | 1.55 | 1.74 | 1.94 | 2.11 | 2.32 | 2.54 | 2.77
      mask TypeOptions pre_emph: 0 | 1 | 2 | 3
      mask TypeOptions post_emph_r2: 0.18 | 0.19 | 0.2 | 0.39 | 0.63 | 0.82 | 1.07 | 1.32 | 1.6 | 1.65 | 1.94 | 2.21 | 2.52 | 2.76 | 3.08 | 3.41 | 3.77 | 3.97 | 4.36 | 4.73 | 5.16 | 5.47 | 5.93 | 6.38 | 6.89
      mask TypeOptions rxeqmix_r2: 0 | 1 | 2 | 3 | 4 | 5 | 6 | 7
      mask TypeOptions swing_r2: 110 | 210 | 310 | 400 | 480 | 570 | 660 | 740 | 810 | 880 | 940 | 990 | 1040 | 1080 | 1110 | 1130
      mask TypeOptions swing: 400 | 500 | 600 | 700 | 800
      mask Callback debug_en_all:
      | if strcmp(get_param(gcb, 'debug_en_all'), 'on')
      |     set_param(gcb, 'debug_dis_all', 'off')
      | end
      mask Callback debug_dis_all:
      | if strcmp(get_param(gcb, 'debug_dis_all'), 'on')
      |     set_param(gcb, 'debug_en_all', 'off')
      | end
      mask Callback txerrctr:
      | blk = gcb;
      | mask_visibilities = get_param(blk, 'MaskVisibilities');
      | mask_names = get_param(blk, 'MaskNames');
      | if strcmp(get_param(blk, 'txerrctr'), 'on')
      |     mask_visibilities{ismember(mask_names, 'txerrctr_len')} = 'on';
      | else
      |     mask_visibilities{ismember(mask_names, 'txerrctr_len')} = 'off';
      | end
      | set_param(blk, 'MaskVisibilities', mask_visibilities);
      mask TypeOptions txsnaplen: 0 - no snap | 256 | 512 | 1024 | 2048 | 4096 | 8192 | 16384
      mask Callback rxerrctr:
      | blk = gcb;
      | mask_visibilities = get_param(blk, 'MaskVisibilities');
      | mask_names = get_param(blk, 'MaskNames');
      | if strcmp(get_param(blk, 'rxerrctr'), 'on')
      |     mask_visibilities{ismember(mask_names, 'rxerrctr_len')} = 'on';
      | else
      |     mask_visibilities{ismember(mask_names, 'rxerrctr_len')} = 'off';
      | end
      | set_param(blk, 'MaskVisibilities', mask_visibilities);
      mask TypeOptions rxsnaplen: 0 - no snap | 256 | 512 | 1024 | 2048 | 4096 | 8192 | 16384
      mask DialogControl ParameterTabVar0 Prompt: Core
      mask DialogControl ParameterTabVar01 Prompt: Debug counters
      mask DialogControl Control2 Prompt: -------------------------------------
      mask DialogControl Control2_copy Prompt: -------------------------------------
  sfp_rst_gpio : xps_library/IO/gpio  Tag=xps:gpio  io_group_params_forwarded=off  io_group=ROACH:led  io_group_real=custom  io_group_custom=qsfp_rst_l  io_dir=out  arith_type=Unsigned  bitwidth=1  bin_pt=0  bit_index=[0]  sample_period=1  use_single_ended=off  use_ddr=off  reg_iob=on  reg_clk_phase=0  termination=None
      settings: SourceProductName=CASPER XPS Blockset
  wires:
  Constant/1 -> onehundred_gbe/7(rx_ack)
  Slice3/1 -> [gbe_stat_rst]
  Slice2/1 -> [gbe_port]
  Slice1/1 -> [gbe_sw_en]
  Slice/1 -> [gbe_sw_rst]
  ctrl/1(in_reg) -> Slice/1, Slice1/1, Slice2/1, Slice3/1
  vld/1 -> Logical/1
  Logical/1 -> onehundred_gbe/3(tx_valid)
  dest_ip/1 -> onehundred_gbe/4(tx_dest_ip)
  eof/1 -> onehundred_gbe/6(tx_end_of_frame), Register/2
  data/1 -> onehundred_gbe/2(tx_data)
  [gbe_sw_rst] -> Delay/1
  Register/1 -> Logical/2
  [gbe_sw_en] -> Register/1
  Delay/1 -> onehundred_gbe/1(rst)
  Constant1/1 -> onehundred_gbe/8(rx_overrun_ack)
  [gbe_stat_rst] -> onehundred_gbe/9(debug_rst)
  byte_enable/1 -> onehundred_gbe/10(tx_byte_enable)
  Constant2/1 -> sfp_rst_gpio/1
  Constant3/1 -> lpmode_gpio/1
  dest_port/1 -> onehundred_gbe/5(tx_dest_port)
